simulink model "untitled1"  (R2023b)
settings: Solver=VariableStepAuto  StartTime=0.0  StopTime=inf  RelTol=1e-3
libraries: ros2lib x3
settings Model: Creator=basten  LastModifiedBy=basten

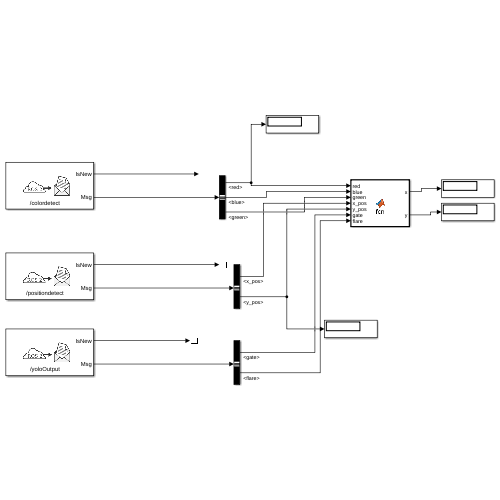
[thumbnail: Simulink's stored preview of the top-level diagram]
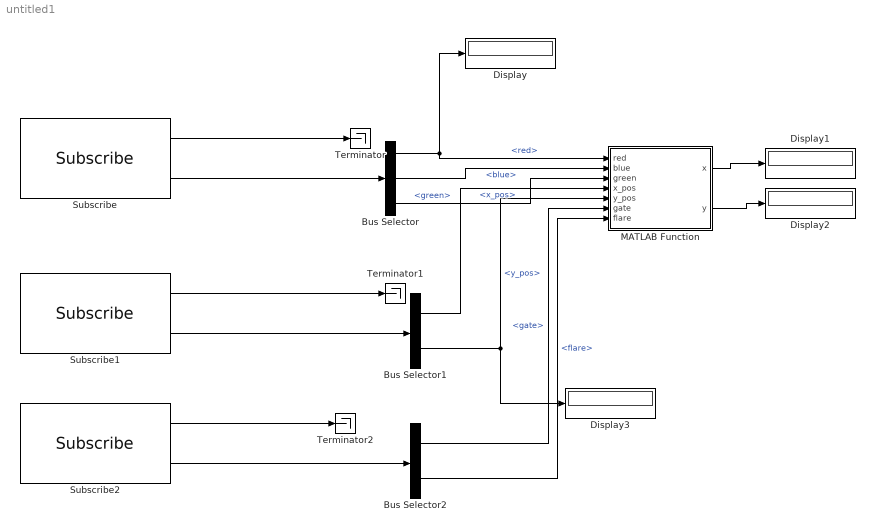
== system untitled1 ==
  Bus Selector : BusSelector  OutputSignals=red,blue,green
  Bus Selector1 : BusSelector  OutputSignals=x_pos,y_pos
  Bus Selector2 : BusSelector  OutputSignals=gate,flare
  Display{,1..3} (4 alike) : Display
  MATLAB Function : MATLAB Function  TreatAsAtomicUnit=on
  Subscribe : ros2lib/Subscribe  topicSource=Specify your own  topic=/colordetect  messageType=tugas_opencv/Color  sampleTime=0.01  QOSHistory=Keep last  QOSDepth=1  QOSReliability=Reliable  QOSDurability=Volatile
  Subscribe1 : ros2lib/Subscribe  topicSource=Specify your own  topic=/positiondetect  messageType=tugas_opencv/Position  sampleTime=0.01  QOSHistory=Keep last  QOSDepth=1  QOSReliability=Reliable  QOSDurability=Volatile
  Subscribe2 : ros2lib/Subscribe  topicSource=Specify your own  topic=/yoloOutput  messageType=tugas_yolo_yolocpp/Seen  sampleTime=0.01  QOSHistory=Keep last  QOSDepth=1  QOSReliability=Reliable  QOSDurability=Volatile
  Terminator : Terminator
  Terminator1 : Terminator
  Terminator2 : Terminator
  wires:
  Subscribe/2 -> Bus Selector/1
  Subscribe/1 -> Terminator/1
  Bus Selector/1 -> Display/1, MATLAB Function/1(red)  "<red>"
  Bus Selector/2 -> MATLAB Function/2(blue)  "<blue>"
  Bus Selector/3 -> MATLAB Function/3(green)  "<green>"
  MATLAB Function/1(x) -> Display1/1
  MATLAB Function/2(y) -> Display2/1
  Subscribe1/1 -> Terminator1/1
  Subscribe1/2 -> Bus Selector1/1
  Bus Selector1/1 -> MATLAB Function/4(x_pos)  "<x_pos>"
  Bus Selector1/2 -> Display3/1, MATLAB Function/5(y_pos)  "<y_pos>"
  Subscribe2/2 -> Bus Selector2/1
  Subscribe2/1 -> Terminator2/1
  Bus Selector2/1 -> MATLAB Function/6(gate)  "<gate>"
  Bus Selector2/2 -> MATLAB Function/7(flare)  "<flare>"

== matlab function untitled1/MATLAB Function ==
  data: x output; red input; y output; blue input; green input; x_pos input; y_pos input; gate input; flare input
function [x, y] = fcn(red, blue, green, x_pos, y_pos, gate, flare)

x = int32(0);
y = int32(0);



persistent currentColor;

if isempty(currentColor)
    currentColor = colorEnum.RED;
end

enumList = enumeration('colorEnum');
currentIndex = find(enumList == currentColor);
currentIndex = currentIndex(1);

nextIndex = mod(currentIndex,3) + 1;

disp(currentIndex);

if currentColor == colorEnum.RED && red
    x = x_pos;
    y = y_pos;
    currentColor = enumList(nextIndex + 1);
end

if currentColor == colorEnum.GREEN && green
    x = x_pos;
    y = y_pos;
    currentColor = enumList(nextIndex + 1);
end

if currentColor == colorEnum.BLUE && blue
    x = x_pos;
    y = y_pos;
    currentColor = enumList(nextIndex + 1);
end
